simulink model "FMrec_J_v2"  (Simulink 9.0)
settings: Solver=FixedStepDiscrete  StartTime=0.0  StopTime=inf  RelTol=1e-3
PreLoadFcn:
  | setenv('MW_MINGW64_LOC','C:\TDM-GCC-64')
StartFcn:
  | tic
StopFcn:
  | toc;
undefined symbols (not defined in the file): magnitude
libraries: dsparch4 x5, UN_HIL_Lib x2, dspobslib x1
Description:
  | QPSK Transmitter and Receiver.
  | 
  | This model shows the implementation of a QPSK transmitter and receiver.
settings Model: FPTRunName=Active  Creator=The MathWorks Inc.  LastModifiedBy=minel
settings DataIOCC: LimitDataPoints=on  SignalLoggingSaveFormat=ModelDataLogs  SaveOutput=off  SaveTime=off
settings OptimizationCC: BooleanDataType=off  DefaultParameterBehavior=Inlined  ExpressionDepthLimit=2147483647  LocalBlockOutputs=off
settings DebuggingCC: AlgebraicLoopMsg=error  SolverPrmCheckMsg=warning  SingleTaskRateTransMsg=error  ParameterPrecisionLossMsg=none  FcnCallInpInsideContextMsg=warning  StateNameClashWarn=warning
settings HardwareCC: TargetBitPerPointer=64  TargetBitPerSizeT=64  TargetBitPerPtrDiffT=64  TargetLongLongMode=on  TargetIntDivRoundTo=Zero  TargetEndianess=LittleEndian  TargetWordSize=64  TargetHWDeviceType=Generic->MATLAB Host Computer  ProdEqTarget=off
settings GRTTargetCC: GeneratePreprocessorConditionals=Disable all
settings ConfigComp: CovSFcnEnable=off
settings SimEventsCC: propDiagStatOutput=1  propPreventDuplicateEvents=0

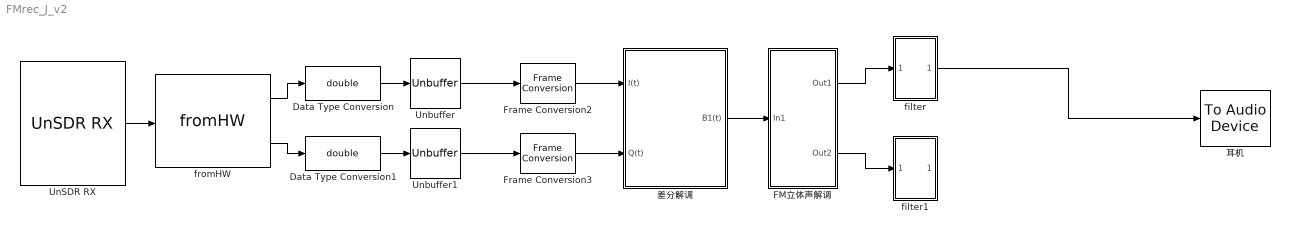
== system FMrec_J_v2 ==
  Data Type Conversion : DataTypeConversion  OutDataTypeStr=double
  Data Type Conversion1 : DataTypeConversion  OutDataTypeStr=double
  FM立体声解调 : Subsystem
  Frame Conversion2 : FrameConversion  InheritSamplingMode=off  OutFrame=Sample-based
  Frame Conversion3 : FrameConversion  InheritSamplingMode=off  OutFrame=Sample-based
  UnSDR RX : UN_HIL_Lib/UnSDR RX  SystemSampleTime=-1
      settings: SourceProductName=HIL Blockset
  Unbuffer : Unbuffer
  Unbuffer1 : Unbuffer
  filter : Subsystem
  filter1 : Subsystem
  fromHW : UN_HIL_Lib/fromHW  sp=1/128000
      settings: SourceProductName=HIL Blockset
  差分解调 : Subsystem
  耳机 : dspobslib/To Audio Device  deviceName=扬声器/听筒 (Realtek Audio)  inheritSampleRate=on  sampleRate=44100  deviceDatatype=Determine from input data type  autoBufferSize=on  bufferSize=4096  queueDuration=2  defaultOutputChannelMapping=on  outputChannelMapping=1:2  outputNumUnderrunSamples=off
      settings: SourceProductName=DSP System Toolbox  SourceProductBaseCode=DS
  wires:
  Unbuffer/1 -> Frame Conversion2/1
  fromHW/1 -> Data Type Conversion/1
  Data Type Conversion/1 -> Unbuffer/1
  fromHW/2 -> Data Type Conversion1/1
  Data Type Conversion1/1 -> Unbuffer1/1
  Unbuffer1/1 -> Frame Conversion3/1
  UnSDR RX/1 -> fromHW/1
  Frame Conversion2/1 -> 差分解调/1(I(t))
  Frame Conversion3/1 -> 差分解调/2(Q(t))
  差分解调/1(B1(t)) -> FM立体声解调/1(In1)
  FM立体声解调/1(Out1) -> filter/1(In1)
  FM立体声解调/2(Out2) -> filter1/1(In1)
  filter/1(Out1) -> 耳机/1

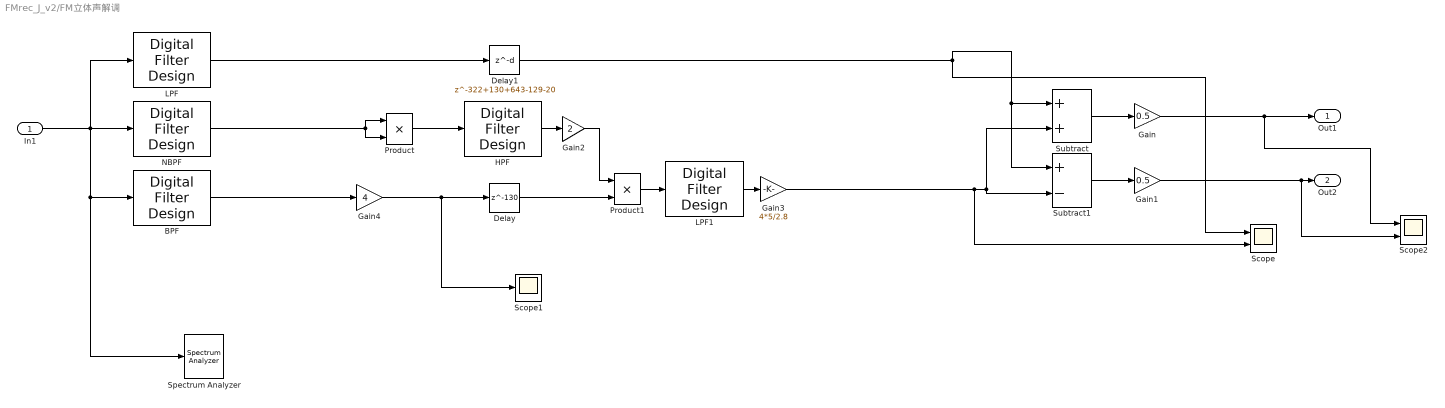
== system FMrec_J_v2/FM立体声解调 ==
  In1 : Inport
  BPF : dsparch4/Digital Filter Design  mwdsp_browser_bugfix_var=off
  Delay : Delay  DelayLength=130  InitialCondition=0
  Delay1 : Delay  DelayLength=322+130+643-129-20  InitialCondition=0
  Gain : Gain  Gain=0.5
  Gain1 : Gain  Gain=0.5
  Gain2 : Gain  Gain=2
  Gain3 : Gain  Gain=4*5/2.8
  Gain4 : Gain  Gain=4
  HPF : dsparch4/Digital Filter Design  mwdsp_browser_bugfix_var=off
  LPF : dsparch4/Digital Filter Design  mwdsp_browser_bugfix_var=off
  LPF1 : dsparch4/Digital Filter Design  mwdsp_browser_bugfix_var=off
  NBPF : dsparch4/Digital Filter Design  mwdsp_browser_bugfix_var=off
  Product : Product
  Product1 : Product
  Scope : Scope  NumInputPorts=2
  Scope1 : Scope
  Scope2 : Scope  NumInputPorts=2
  Spectrum Analyzer : SpectrumAnalyzer
  Subtract : Sum
  Subtract1 : Sum  Inputs=+-
  Out1 : Outport
  Out2 : Outport  Port=2
  wires:
  HPF/1 -> Gain2/1
  Product1/1 -> LPF1/1
  LPF1/1 -> Gain3/1
  Gain2/1 -> Product1/1
  LPF/1 -> Delay1/1
  Product/1 -> HPF/1
  Subtract/1 -> Gain/1
  Gain1/1 -> Scope2/2, Out2/1
  Subtract1/1 -> Gain1/1
  Gain/1 -> Scope2/1, Out1/1
  BPF/1 -> Gain4/1
  Delay/1 -> Product1/2
  In1/1 -> LPF/1, Spectrum Analyzer/1, BPF/1, NBPF/1
  NBPF/1 -> Product/2, Product/1
  Gain4/1 -> Scope1/1, Delay/1
  Delay1/1 -> Subtract1/1, Subtract/1, Scope/1
  Gain3/1 -> Subtract/2, Subtract1/2, Scope/2

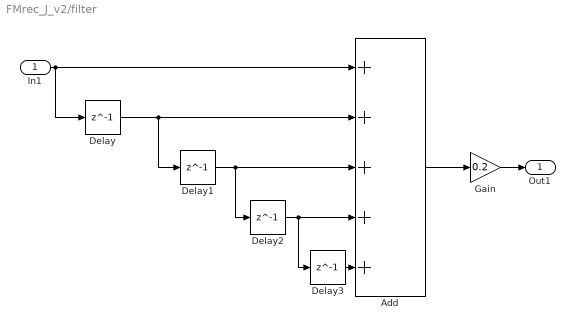
== system FMrec_J_v2/filter ==
  In1 : Inport
  Add : Sum  Inputs=+++++
  Delay{,1..3} (4 alike) : Delay  DelayLength=1  InitialCondition=0
  Gain : Gain  Gain=0.2
  Out1 : Outport
  wires:
  In1/1 -> Add/1, Delay/1
  Add/1 -> Gain/1
  Gain/1 -> Out1/1
  Delay/1 -> Delay1/1, Add/2
  Delay1/1 -> Delay2/1, Add/3
  Delay2/1 -> Delay3/1, Add/4
  Delay3/1 -> Add/5

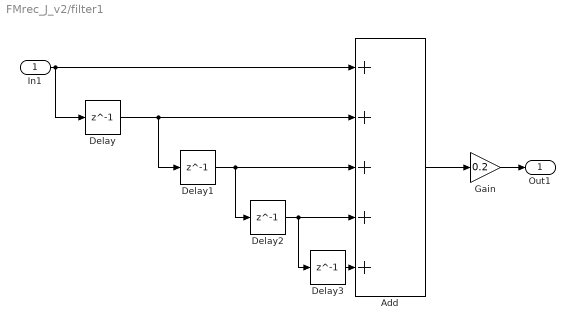
== system FMrec_J_v2/filter1 ==
  In1 : Inport
  Add : Sum  Inputs=+++++
  Delay{,1..3} (4 alike) : Delay  DelayLength=1  InitialCondition=0
  Gain : Gain  Gain=0.2
  Out1 : Outport
  wires:
  In1/1 -> Add/1, Delay/1
  Add/1 -> Gain/1
  Gain/1 -> Out1/1
  Delay/1 -> Delay1/1, Add/2
  Delay1/1 -> Delay2/1, Add/3
  Delay2/1 -> Delay3/1, Add/4
  Delay3/1 -> Add/5

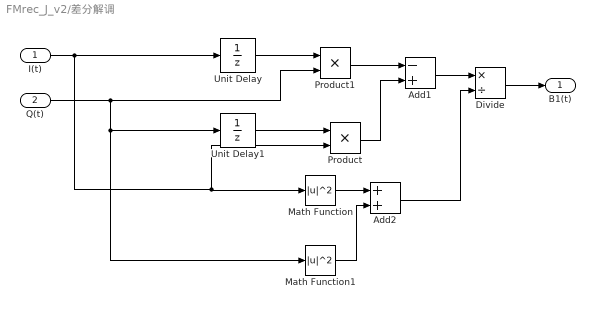
== system FMrec_J_v2/差分解调 ==
  I(t) : Inport
  Q(t) : Inport  Port=2
  Add1 : Sum  Inputs=-+
  Add2 : Sum
  Divide : Product  Inputs=*/
  Math Function : Math  Operator=magnitude^2  SaturateOnIntegerOverflow=on
  Math Function1 : Math  Operator=magnitude^2  SaturateOnIntegerOverflow=on
  Product : Product  RndMeth=Zero
  Product1 : Product  RndMeth=Zero
  Unit Delay : UnitDelay  SampleTime=-1
  Unit Delay1 : UnitDelay  SampleTime=-1
  B1(t) : Outport
  wires:
  Add1/1 -> Divide/1
  Add2/1 -> Divide/2
  Product/1 -> Add1/2
  Product1/1 -> Add1/1
  Unit Delay/1 -> Product1/1
  Unit Delay1/1 -> Product/1
  Q(t)/1 -> Math Function1/1, Unit Delay1/1, Product1/2
  I(t)/1 -> Product/2, Math Function/1, Unit Delay/1
  Math Function/1 -> Add2/1
  Math Function1/1 -> Add2/2
  Divide/1 -> B1(t)/1
